simulink model "rayleighfading"  (Simulink 6.0)
settings: Solver=ode45  StartTime=0.0  StopTime=Inf  RelTol=1e-3
undefined symbols (not defined in the file or in its folder): slcm
libraries: commchan2 x1, commdigbbndpm2 x1, commsink2 x1, commfilt2 x1, commrandsrc2 x1
CloseFcn:
  | clear rayleighSigsOut
settings Model: Creator=mclune  LastModifiedBy=fwei  BufferReuse=off
settings DataIOCC: LimitDataPoints=off  SaveOutput=off  SaveTime=off  SignalLoggingName=rayleighSigsOut
settings OptimizationCC: BooleanDataType=off  OptimizeBlockIOStorage=off  BufferReuse=off  LocalBlockOutputs=off
settings DebuggingCC: CheckExecutionContextPreStartOutputMsg=on  CheckExecutionContextRuntimeOutputMsg=on  SolverPrmCheckMsg=none
settings HardwareCC: TargetUnknown=on
settings ModelReferenceCC: UpdateModelReferenceTargets=IfOutOfDate
settings GRTTargetCC: LifeSpan=inf
settings SFSimCC: SFSimApplyToAllLibs=on  SFSimBuildMode=Incremental

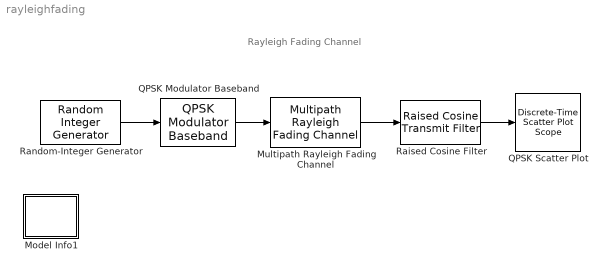
== system rayleighfading ==
  note: Rayleigh Fading Channel
  Model Info1 : Subsystem  LoadFcn=slcm LoadBlock;  InitFcn=slcm('UpdateAllCMBlocksInThisModelInit')  EnableExecutionContextPropagation=on  mask(CMBlock){InitialSaveTempField=, InitialBlockCM=None, BlockCM=None, Frame=on, SaveTempField=, DisplayStringWithTags=Info, MaskDisplayString=Info, HorizontalTextAlignment=Center, LeftAlignmentValue=0.5, SourceBlockDiagram=rayleighfading, TagMaxNumber=20, CMTag1=, CMTag2=, CMTag3=, CMTag4=, CMTag5=, CMTag6=, CMTag7=, CMTag8=, CMTag9=, CMTag10=, CMTag11=, CMTag12=, CMTag13=, CMTag14=, CMTag15=, CMTag16=, CMTag17=, CMTag18=, CMTag19=, CMTag20=}
      mask help: This block allows revision control information to be displayed within the model.
      settings: CopyFcn=slcm CopyBlock;  DeleteFcn=slcm Cancel;  PostSaveFcn=slcm('UpdateAllCMBlocksInThisModel')  NameChangeFcn=slcm Rename;  OpenFcn=commdemohelp;
      mask Display: text(str2num(LeftAlignmentValue), 0.5, MaskDisplayString, 'HorizontalAlignment', HorizontalTextAlignment)
  Multipath Rayleigh Fading Channel : commchan2/Multipath Rayleigh Fading Channel  Fd=40  simTs=1e-5  delayVec=[0 2e-5]  gainVecdB="[0  -9 ]"  normGain=on  Seed=12345
  QPSK Modulator Baseband : commdigbbndpm2/QPSK Modulator Baseband  InType=Integer  Enc=Binary  Ph=pi/4  numSamp=1
  QPSK Scatter Plot : commsink2/Discrete-Time Scatter Plot Scope  Tag=ScatterPlot  sampPerSymb=8  offsetEye=0  numTraces=40  numNewFrames=10  LineMarkers=.  LineColors=b  fading=on  render=on  AxisGrid=on  xMin=-1.5  xMax=1.5  yMin=-1.5  yMax=1.5  inphaseLabel=In-phase Amplitude  quadratureLabel=Quadrature Amplitude  openScopeAtSimStart=on  FrameNumber=off  FigPos=[26 333 358 358]  figTitle=Scatter Plot  numLinesMax=50  block_type_=scatter
  Raised Cosine Filter : commfilt2/Raised Cosine Transmit Filter  filtType=Normal  D=2  R=0.3  sampMode=Frame-based  N=8  checkGain=Normalized  filterGain=1  checkCoeff=off  variableName=rcTxFilt  launchFVT=off
  Random-Integer Generator : commrandsrc2/Random Integer Generator  mul=4  seed=[12345]  Ts=1e-5  frameBased=on  sampPerFrame=50  orient=off
  wires:
  Random-Integer Generator/1 -> QPSK Modulator Baseband/1
  QPSK Modulator Baseband/1 -> Multipath Rayleigh Fading Channel/1
  Multipath Rayleigh Fading Channel/1 -> Raised Cosine Filter/1
  Raised Cosine Filter/1 -> QPSK Scatter Plot/1

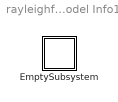
== system rayleighfading/Model Info1 ==
  EmptySubsystem : Subsystem  EnableExecutionContextPropagation=on

== system rayleighfading/Model Info1/EmptySubsystem ==
